simulink model "enabled_subsystem_example"  (R2019b)
settings: Solver=FixedStepDiscrete  StartTime=0.0  StopTime=10  RelTol=1e-3
settings Model: Creator=svanbeek  LastModifiedBy=bhisma
settings DataIOCC: LimitDataPoints=on  SaveFormat=Array  SaveOutput=off  SignalLogging=off  SaveTime=off  ReturnWorkspaceOutputs=off
settings OptimizationCC: BlockReduction=off  ConditionallyExecuteInputs=off  DefaultParameterBehavior=Inlined  ExpressionDepthLimit=2147483647  LifeSpan=inf
settings DebuggingCC: AlgebraicLoopMsg=error  UnderspecifiedInitializationDetection=Classic  MergeDetectMultiDrivingBlocksExec=none  SolverPrmCheckMsg=warning  SingleTaskRateTransMsg=error  StateNameClashWarn=warning  SFUnexpectedBacktrackingDiag=warning  SFNoUnconditionalDefaultTransitionDiag=warning  SFExecutionAtInitializationDiag=none  ArithmeticOperatorsInVariantConditions=warning
settings HardwareCC: ProdBitPerPointer=32  ProdBitPerSizeT=32  ProdBitPerPtrDiffT=32  ProdLargestAtomicFloat=None  ProdIntDivRoundTo=Undefined  ProdEndianess=Unspecified  ProdWordSize=32  ProdHWDeviceType=ASIC/FPGA->ASIC/FPGA  ProdEqTarget=off
settings ModelReferenceCC: PropagateSignalLabelsOutOfModel=off
settings SFSimCC: SimUseLocalCustomCode=off  CustomCodeUndefinedFunction=UseInterfaceOnly
settings RTWCC: RTWUseLocalCustomCode=off
settings CodeAppCC: StateflowObjectComments=on
settings GRTTargetCC: TargetLangStandard=C89/C90 (ANSI)  GeneratePreprocessorConditionals=Disable all
settings ConfigComp: CovMetricSettings=dw  CovHtmlReporting=on  CovSaveCumulativeToWorkspaceVar=on  CovSaveSingleToWorkspaceVar=on  CovExternalEMLEnable=off  CovSFcnEnable=off

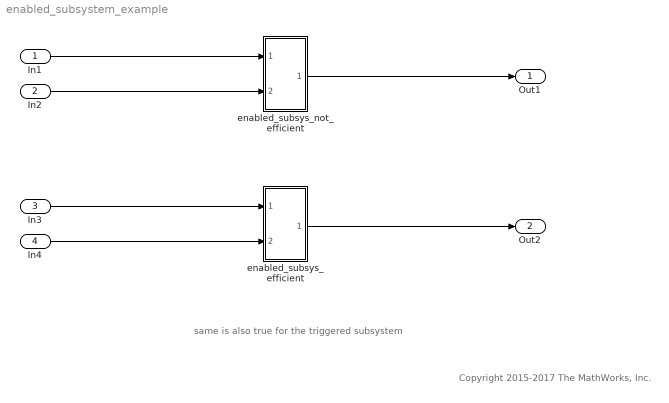
== system enabled_subsystem_example ==
  note: Copyright 2015-2017 The MathWorks, Inc.
  note: same is also true for the triggered subsystem
  In1 : Inport  OutDataTypeStr=fixdt(1,16,14)  SampleTime=1
  In2 : Inport  Port=2  OutDataTypeStr=boolean  SampleTime=1
  In3 : Inport  Port=3  OutDataTypeStr=fixdt(1,16,14)  SampleTime=1
  In4 : Inport  Port=4  OutDataTypeStr=boolean  SampleTime=1
  enabled_subsys_efficient : Subsystem
  enabled_subsys_not_efficient : Subsystem
  Out1 : Outport
  Out2 : Outport  Port=2
  wires:
  In1/1 -> enabled_subsys_not_efficient/1(In1)
  enabled_subsys_not_efficient/1(Out1) -> Out1/1
  In2/1 -> enabled_subsys_not_efficient/2(In2)
  In3/1 -> enabled_subsys_efficient/1(In1)
  enabled_subsys_efficient/1(Out1) -> Out2/1
  In4/1 -> enabled_subsys_efficient/2(In2)

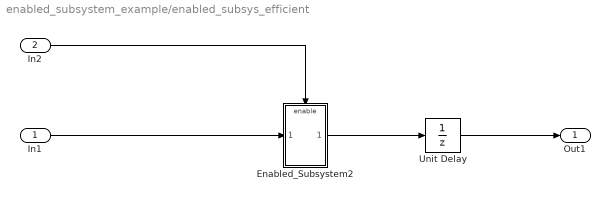
== system enabled_subsystem_example/enabled_subsys_efficient ==
  In1 : Inport
  In2 : Inport  Port=2
  Enabled_Subsystem2 : Subsystem  Description=|
      | the unit delay will be absorbed by the enabled subsystem
      | but no bypass register and mux will be needed anymore
      settings: AttributesFormatString=%<Description>
  Unit Delay : UnitDelay  SampleTime=-1  HasFrameUpgradeWarning=on
  Out1 : Outport
  wires:
  In2/1 -> Enabled_Subsystem2/Enable
  Enabled_Subsystem2/1(Out1) -> Unit Delay/1
  In1/1 -> Enabled_Subsystem2/1(In1)
  Unit Delay/1 -> Out1/1

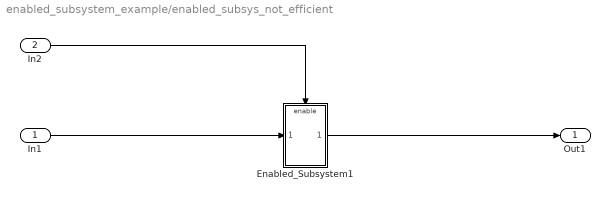
== system enabled_subsystem_example/enabled_subsys_not_efficient ==
  In1 : Inport
  In2 : Inport  Port=2
  Enabled_Subsystem1 : Subsystem  Description=this will result in a bypass register and mux
      settings: AttributesFormatString=%<Description>
  Out1 : Outport
  wires:
  In1/1 -> Enabled_Subsystem1/1(In1)
  Enabled_Subsystem1/1(Out1) -> Out1/1
  In2/1 -> Enabled_Subsystem1/Enable

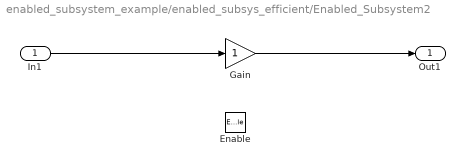
== system enabled_subsystem_example/enabled_subsys_efficient/Enabled_Subsystem2 ==
  In1 : Inport
  Enable : EnablePort
  Gain : Gain
  Out1 : Outport  InitialOutput=0
  wires:
  In1/1 -> Gain/1
  Gain/1 -> Out1/1

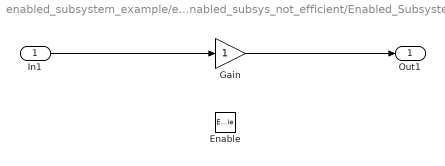
== system enabled_subsystem_example/enabled_subsys_not_efficient/Enabled_Subsystem1 ==
  In1 : Inport
  Enable : EnablePort
  Gain : Gain
  Out1 : Outport  InitialOutput=0
  wires:
  Gain/1 -> Out1/1
  In1/1 -> Gain/1
